simulink model "TEG_ESC_Benchmark"  (R2021b)
settings: Solver=VariableStepAuto  StartTime=0.0  StopTime=0.1  RelTol=1e-3  EnableMultiTasking=on
values from neighbouring files (symbols this model uses):
  delta_T = Th - Tc    (= 380)    [TEG_BenchmarkStart.m]
  m = 1    [TEG_BenchmarkStart.m]
  RL = (Vm^2)/Wm    (= 7.2)    [TEG_BenchmarkStart.m]
  Tc = Tc + 273.15    (= 293.15)    [TEG_BenchmarkStart.m]
  Th = Th + 273.15    (= 673.15)    [TEG_BenchmarkStart.m]
  Vm = 1.2    [TEG_BenchmarkStart.m]
  Wm = 0.2    [TEG_BenchmarkStart.m]
undefined symbols (not defined in the file or in its folder): Ion, Lithium
libraries: spsSeriesRLCBranchLib x3, spsCurrentMeasurementLib x2, simulink x2, spsVoltageMeasurementLib x2, spsBatteryLib x1, spsControlledVoltageSourceLib x1, spsDiodeLib x1, slctrlblks x1, spsMeanLib x1, spsPWMGeneratorDCDCLib x1, spsMosfetLib x1, spspowerguiLib x1
settings Model: Creator=Hadi  LastModifiedBy=romem
settings SolverCC: ZeroCrossAlgorithm=Adaptive  AlgebraicLoopSolver=TrustRegion
settings DataIOCC: LimitDataPoints=on  SaveFormat=Array  SignalLoggingSaveFormat=ModelDataLogs  ReturnWorkspaceOutputs=off
settings OptimizationCC: ExpressionDepthLimit=2147483647  LifeSpan=inf
settings DebuggingCC: UnderspecifiedInitializationDetection=Classic  MergeDetectMultiDrivingBlocksExec=none  IgnoredZcDiagnostic=none  SolverPrmCheckMsg=warning  FcnCallInpInsideContextMsg=warning  StateNameClashWarn=warning  SFUnexpectedBacktrackingDiag=warning  SFNoUnconditionalDefaultTransitionDiag=warning  SFExecutionAtInitializationDiag=none  SFMachineParentedDataDiag=warning  ArithmeticOperatorsInVariantConditions=warning
settings HardwareCC: ProdBitPerPointer=32  ProdBitPerSizeT=32  ProdBitPerPtrDiffT=32  ProdLargestAtomicFloat=None  ProdIntDivRoundTo=Undefined  ProdEndianess=Unspecified  ProdWordSize=32  ProdHWDeviceType=32-bit Generic  TargetBitPerPointer=64  TargetBitPerSizeT=64  TargetBitPerPtrDiffT=64  TargetLongLongMode=on  TargetIntDivRoundTo=Zero  TargetEndianess=LittleEndian  TargetWordSize=64  TargetHWDeviceType=MATLAB Host  ProdEqTarget=off
settings ModelReferenceCC: PropagateSignalLabelsOutOfModel=off
settings SFSimCC: SimUseLocalCustomCode=off  CustomCodeUndefinedFunction=UseInterfaceOnly
settings RTWCC: Description=S-function Target  SystemTargetFile=rtwsfcn.tlc  TemplateMakefile=rtwsfcn_default_tmf  RTWUseLocalCustomCode=off
settings CodeAppCC: StateflowObjectComments=on
settings STFCustomTargetCC: ModelReferenceCompliant=off  CompOptLevelCompliant=on  MATLABClassNameForMDSCustomization=Simulink.SoftwareTarget.TargetSpecificTriggerConfigurationBase  SystemTargetFile=rtwsfcn.tlc
settings ConfigComp: CovMetricSettings=dw  CovSaveCumulativeToWorkspaceVar=on  CovSaveSingleToWorkspaceVar=on  CovExternalEMLEnable=off

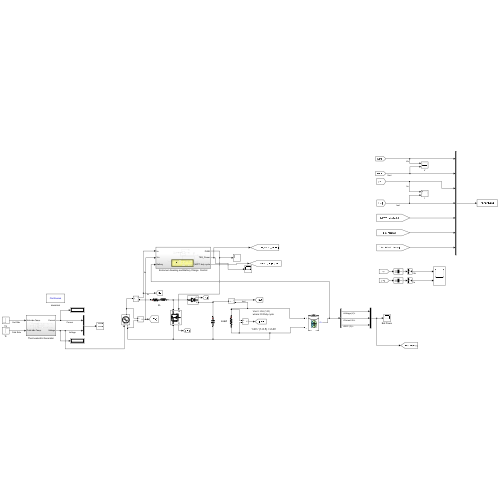
[thumbnail: Simulink's stored preview of the top-level diagram]
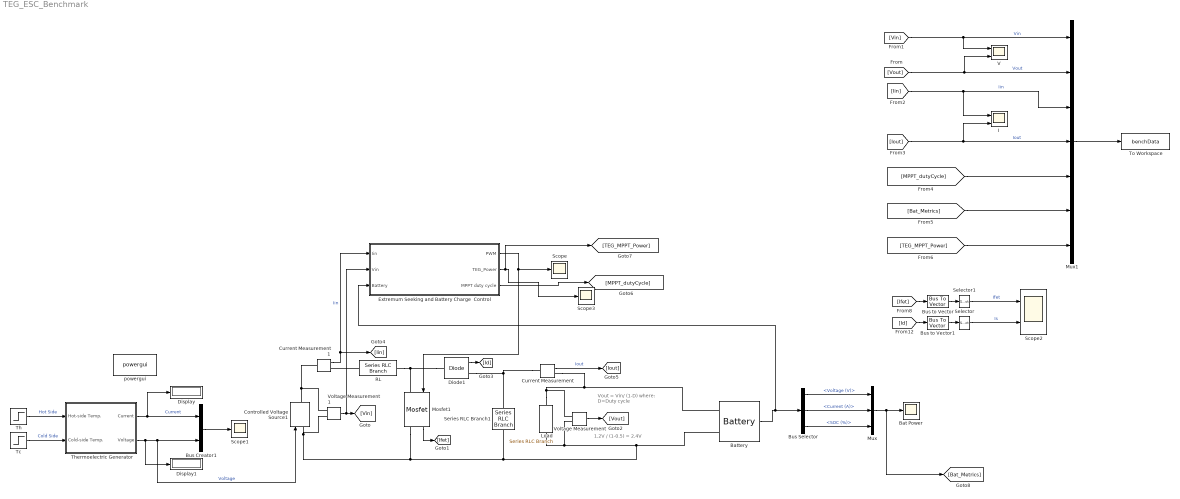
== system TEG_ESC_Benchmark ==
  note: Vout = Vin/ (1-D)
      | where: D=Duty cycle
  note: 1.2V / (1-0.5) = 2.4V
  Bat Power : Scope
  Battery : spsBatteryLib/Battery  BatType=Lithium-Ion  ShowTempParam=off  ThermalPreset="3.7V  4.4Ah"  ShowAgeParam=off  NomV=3.4  NomQ=4.4  SOC=10  Batt_Tr=5  PresetModel=off  MaxQ=4.5  MinV=2.55  FullV=4.125  Dis_rate=0.9  R=0.00818  Normal_OP=4  expZone="[4         0.5]"  current=[6.5 13 32.5]  Units=Time  Tci=20  NomT=20  T2=-30  MaxQ2=3.8  FullV2=3.38  Normal_OP2=2.75  expZone2="[3.25         0.5]"  Rca=0.06  ti=1000  Dp=0  Neq0=0  Tsim=1e6  Ta1=25  Qeol=5.4*0.9  Reol=0.013333*1.2  Char_age=[2.3478, 3]  Dis_age=[2.3478, 10]  N1=1500  N2=10500  N3=1000  N4=1400  Ta2=45  N5=950
  Bus Creator1 : BusCreator  Inputs=2
  Bus Selector : BusSelector  OutputSignals=Voltage (V),Current (A),SOC (%)
  Bus to Vector : BusToVector
  Bus to Vector1 : BusToVector
  Controlled Voltage Source1 : spsControlledVoltageSourceLib/Controlled Voltage Source  Initialize=on  Source_Type=DC  Amplitude=0  Phase=0  Frequency=0  Measurements=None
  Current Measurement : spsCurrentMeasurementLib/Current Measurement  PhasorSimulation=off  OutputType=Complex  PSBequivalent=0
  Current Measurement1 : spsCurrentMeasurementLib/Current Measurement  PhasorSimulation=off  OutputType=Complex  PSBequivalent=0
  Diode1 : spsDiodeLib/Diode  Ron=1e-3  Lon=0  Vf=0  IC=0  UseSnubber=off  Rs=inf  Cs=inf  Measurements=on
  Display : Display
  Display1 : Display
  Extremum Seeking and Battery Charge  Control : Subsystem
  I : Scope  NumInputPorts=2
  Load : spsSeriesRLCBranchLib/Series RLC Branch  LConnTagsString=__new0  RConnTagsString=__new0  BranchType=R  Resistance=100  Inductance=200e-6  SetiL0=off  InitialCurrent=0  Capacitance=400e-6  Setx0=off  InitialVoltage=0  Measurements=None
  Mosfet1 : spsMosfetLib/Mosfet  Ron=1e-3  Lon=0  Rd=1e-3  Vfd=0  IC=0  Rs=inf  Cs=inf  Measurements=on
  Mux : Mux  Inputs=3
  Mux1 : Mux  Inputs=7
  RL : spsSeriesRLCBranchLib/Series RLC Branch  LConnTagsString=__new0  RConnTagsString=__new0  BranchType=RL  Resistance=1e-3  Inductance=250e-6  SetiL0=off  InitialCurrent=0  Capacitance=1e-6  Setx0=off  InitialVoltage=0  Measurements=None
  Scope : Scope
  Scope1 : Scope
  Scope2 : Scope  NumInputPorts=2
  Scope3 : Scope
  Selector : Selector  InputPortWidth=2  IndexOptions=Index vector (dialog)  Indices=1  OutputSizes=1
  Selector1 : Selector  InputPortWidth=2  IndexOptions=Index vector (dialog)  Indices=1  OutputSizes=1
  Series RLC Branch1 : spsSeriesRLCBranchLib/Series RLC Branch  LConnTagsString=__new0  RConnTagsString=__new0  BranchType=C  Resistance=1e-4  Inductance=200e-6  SetiL0=off  InitialCurrent=0  Capacitance=200e-6  Setx0=off  InitialVoltage=40  Measurements=None
  Tc : Step  Time=0  After=Tc  SampleTime=0
  Th : Step  Time=0  After=Th  SampleTime=0
  Thermoelectric Generator : Subsystem
  To Workspace : ToWorkspace  VariableName=benchData  SaveFormat=Timeseries  SampleTime=-1
  V : Scope  NumInputPorts=2
  Voltage Measurement : spsVoltageMeasurementLib/Voltage Measurement  PhasorSimulation=off  OutputType=Complex  PSBequivalent=0
  Voltage Measurement1 : spsVoltageMeasurementLib/Voltage Measurement  PhasorSimulation=off  OutputType=Complex  PSBequivalent=0
  powergui : spspowerguiLib/powergui  Priority=1  SimulationMode=Continuous  SampleTime=50e-6  frequency=60  Iterations=50  frequencyindice=0  Pbase=100e6  ErrMax=1e-4  UnitsV=kV  UnitsW=MW  buscounter=0  FunctionMessages=off  echomessages=off  EnableUseOfTLC=off  CurrentSourceSwitches=off  DisableSnubberDevices=off  DisableRonSwitches=off  DisableVfSwitches=off  DisplayEquations=off  AutomaticDiscreteSolvers=off  SolverType=Tustin/Backward Euler (TBE)  Interpol=off  ExternalGateDelay=off  methode=off  Ts=100  x0status=blocks  SPID=on  SwTol=0  HookPort=off  NonlinearTolerance=1e-4  nMaxIteration=100  ContinueOnMaxIteration=off  RestoreLinks=warning  ResistiveCurrentMeasurement=off  Frange=[0:2:500]  Ylog=off  Xlog=on  ShowGrid=off  save=off  variable=ZData  structure=0  ZoomFFT=off  StartTime=0.0  cycles=1  DisplayStyle=1  fundamental=60  FreqAxis=off  MaxFrequency=1000  frequencyindicesteady=1  RmsSteady=1  display=off
  wires:
  Bus Selector/2 -> Mux/2  "<Current (A)>"
  Current Measurement/1 -> [Iout]  "Iout"
  Diode1/1 -> [Id]
  Voltage Measurement1/1 -> Extremum Seeking and Battery Charge  Control/2(Vin), [Vin]
  Voltage Measurement/1 -> [Vout]
  Tc/1 -> Thermoelectric Generator/2(Cold-side Temp.)  "Cold Side"
  Thermoelectric Generator/1(Current) -> Display/1, Bus Creator1/1  "Current"
  Bus Selector/3 -> Mux/3  "<SOC (%)>"
  Battery/1 -> Extremum Seeking and Battery Charge  Control/3(Battery), Bus Selector/1
  Current Measurement1/1 -> Extremum Seeking and Battery Charge  Control/1(Iin), [Iin]  "Iin"
  Mux/1 -> [Bat_Metrics], Bat Power/1
  Th/1 -> Thermoelectric Generator/1(Hot-side Temp.)  "Hot Side"
  Bus Selector/1 -> Mux/1  "<Voltage (V)>"
  Mosfet1/1 -> [Ifet]
  Thermoelectric Generator/2(Voltage) -> Display1/1, Bus Creator1/2, Controlled Voltage Source1/1  "Voltage"
  Bus Creator1/1 -> Scope1/1
  Extremum Seeking and Battery Charge  Control/1(PWM) -> Scope/1, Mosfet1/1
  Selector1/1 -> Scope2/1  "Ifet"
  [Vout] -> V/2, Mux1/2  "Vout"
  Bus to Vector/1 -> Selector1/1
  [Vin] -> V/1, Mux1/1  "Vin"
  Mux1/1 -> To Workspace/1
  [MPPT_dutyCycle] -> Mux1/5
  [Ifet] -> Bus to Vector/1
  Bus to Vector1/1 -> Selector/1
  [Iin] -> Mux1/3, I/1  "Iin"
  Selector/1 -> Scope2/2  "Is"
  [Bat_Metrics] -> Mux1/6
  [TEG_MPPT_Power] -> Mux1/7
  [Iout] -> I/2, Mux1/4  "Iout"
  [Id] -> Bus to Vector1/1
  Extremum Seeking and Battery Charge  Control/2(TEG_Power) -> [TEG_MPPT_Power], Scope3/1
  Extremum Seeking and Battery Charge  Control/3(MPPT duty cycle) -> [MPPT_dutyCycle]
  connections:
  Current Measurement1/LConn1 -- Voltage Measurement1/LConn1 -- Controlled Voltage Source1/RConn1
  Mosfet1/RConn1 -- Load/RConn1 -- Voltage Measurement/LConn2 -- Battery/LConn2 -- Series RLC Branch1/RConn1 -- Voltage Measurement1/LConn2 -- Controlled Voltage Source1/LConn1
  Diode1/LConn1 -- RL/RConn1 -- Mosfet1/LConn1
  Current Measurement/LConn1 -- Series RLC Branch1/LConn1 -- Diode1/RConn1
  Load/LConn1 -- Voltage Measurement/LConn1 -- Battery/LConn1 -- Current Measurement/RConn1
  RL/LConn1 -- Current Measurement1/RConn1

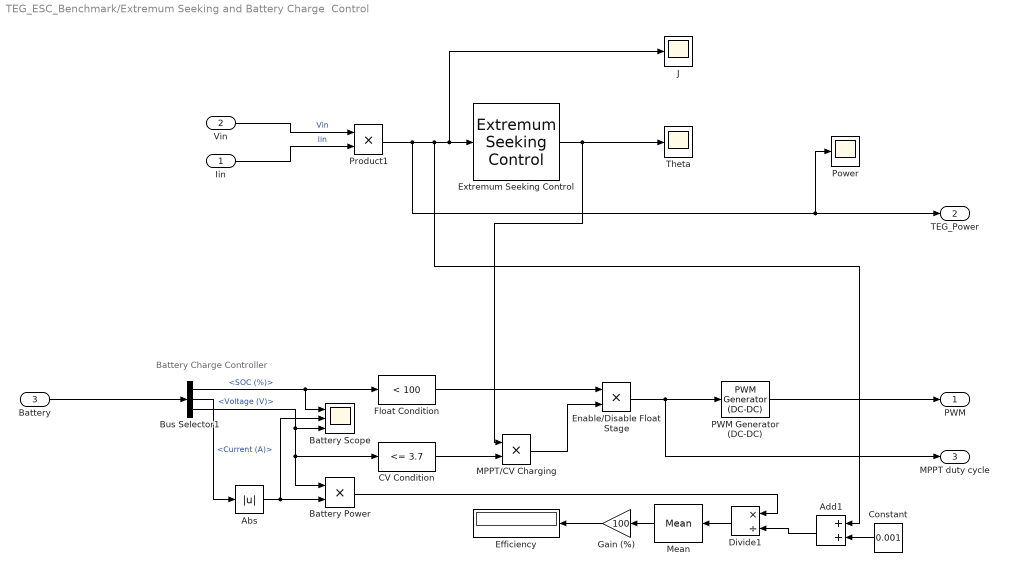
== system TEG_ESC_Benchmark/Extremum Seeking and Battery Charge  Control ==
  note: Battery Charge Controller
  Iin : Inport
  Vin : Inport  Port=2
  Battery : Inport  Port=3
  Abs : Abs
  Add1 : Sum
  Battery Power : Product
  Battery Scope : Scope  NumInputPorts=3
  Bus Selector1 : BusSelector  OutputSignals=SOC (%),Current (A),Voltage (V)
  CV Condition : simulink/Logic and Bit Operations/Compare To Constant  relop=<=  const=3.7  OutDataTypeStr=boolean
  Constant : Constant  Value=0.001
  Divide1 : Product  Inputs=*/
  Efficiency : Display
  Enable/Disable Float Stage : Product
  Extremum Seeking Control : slctrlblks/Extremum Seeking Control  timeDomainStatus=Continuous time  SampleTime=0.1  IntegratorMethods=Forward Euler  paramCount=1  initialVal=0  omega=1  gain=1  demodAmp=1  demodPhase=0  modAmp=0.1  modPhase=0  highPassEnable=off  highPassCutoff=1  lowPassEnable=off  lowPassCutoff=1  estimatedVarOn=off  HPFFreq=1  LPFFreq=1  SampleTimeVar=0
      settings: SourceProductBaseCode=SD
  Float Condition : simulink/Logic and Bit Operations/Compare To Constant  relop=<  const=100  OutDataTypeStr=boolean
  Gain (%) : Gain  Gain=100
  J : Scope
  MPPT/CV Charging : Product
  Mean : spsMeanLib/Mean  Freq=1  Vinit=0  Ts=0
      link override Model/integrator: InitialCondition=0
  PWM Generator (DC-DC) : spsPWMGeneratorDCDCLib/PWM Generator (DC-DC)  Fsw=20e3  Ts=0
  Power : Scope
  Product1 : Product  RndMeth=Zero
  Theta : Scope
  PWM : Outport  VectorParamsAs1DForOutWhenUnconnected=off
  TEG_Power : Outport  Port=2  VectorParamsAs1DForOutWhenUnconnected=off
  MPPT duty cycle : Outport  Port=3  VectorParamsAs1DForOutWhenUnconnected=off
  wires:
  Vin/1 -> Product1/1  "Vin"
  Iin/1 -> Product1/2  "Iin"
  CV Condition/1 -> MPPT/CV Charging/2
  PWM Generator (DC-DC)/1 -> PWM/1
  Bus Selector1/3 -> Battery Scope/3, CV Condition/1, Battery Power/1  "<Voltage (V)>"
  Mean/1 -> Gain (%)/1
  Bus Selector1/2 -> Abs/1  "<Current (A)>"
  MPPT/CV Charging/1 -> Enable/Disable Float Stage/2
  Bus Selector1/1 -> Float Condition/1, Battery Scope/1  "<SOC (%)>"
  Divide1/1 -> Mean/1
  Float Condition/1 -> Enable/Disable Float Stage/1
  Constant/1 -> Add1/2
  Abs/1 -> Battery Scope/2, Battery Power/2
  Gain (%)/1 -> Efficiency/1
  Battery Power/1 -> Divide1/1
  Enable/Disable Float Stage/1 -> MPPT duty cycle/1, PWM Generator (DC-DC)/1
  Extremum Seeking Control/1 -> MPPT/CV Charging/1, Theta/1
  Battery/1 -> Bus Selector1/1
  Add1/1 -> Divide1/2
  Product1/1 -> Power/1, TEG_Power/1, Add1/1, J/1, Extremum Seeking Control/1

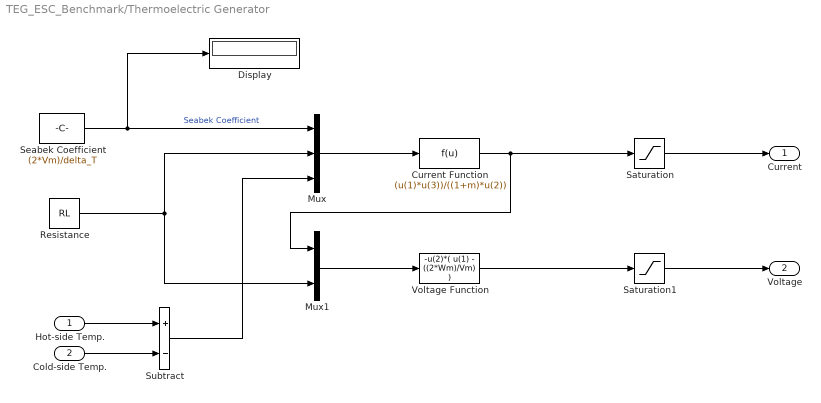
== system TEG_ESC_Benchmark/Thermoelectric Generator ==
  Hot-side Temp. : Inport
  Cold-side Temp. : Inport  Port=2
  Current Function : Fcn  Expr=(u(1)*u(3))/((1+m)*u(2))
  Display : Display
  Mux : Mux  Inputs=3
  Mux1 : Mux  Inputs=2
  Resistance : Constant  Value=RL
  Saturation : Saturate  UpperLimit=0.170  LowerLimit=0
  Saturation1 : Saturate  UpperLimit=1.2  LowerLimit=0
  Seabek Coefficient : Constant  Value=(2*Vm)/delta_T
  Subtract : Sum  Inputs=+-
  Voltage Function : Fcn  Expr=-u(2)*( u(1) - ((2*Wm)/Vm) )
  Current : Outport  VectorParamsAs1DForOutWhenUnconnected=off
  Voltage : Outport  Port=2  VectorParamsAs1DForOutWhenUnconnected=off
  wires:
  Hot-side Temp./1 -> Subtract/1
  Cold-side Temp./1 -> Subtract/2
  Current Function/1 -> Saturation/1, Mux1/1
  Mux1/1 -> Voltage Function/1
  Resistance/1 -> Mux1/2, Mux/2
  Seabek Coefficient/1 -> Display/1, Mux/1  "Seabek Coefficient"
  Subtract/1 -> Mux/3
  Mux/1 -> Current Function/1
  Saturation/1 -> Current/1
  Voltage Function/1 -> Saturation1/1
  Saturation1/1 -> Voltage/1
